simulink model "dcm2quat_test"  (R2018b)
settings: Solver=VariableStepAuto  StartTime=0.0  StopTime=10.0  RelTol=1e-3
libraries: sharedtransform x1
settings Model: Creator=taylorreynolds  LastModifiedBy=taylorreynolds

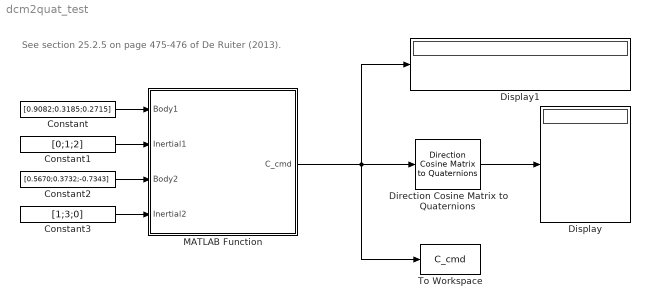
== system dcm2quat_test ==
  note: See section 25.2.5 on page 475-476 of De Ruiter (2013).
  Constant : Constant  Value=[0.9082;0.3185;0.2715]
  Constant1 : Constant  Value=[0;1;2]
  Constant2 : Constant  Value=[0.5670;0.3732;-0.7343]
  Constant3 : Constant  Value=[1;3;0]
  Direction Cosine Matrix to Quaternions : sharedtransform/Direction Cosine Matrix  to Quaternions  aMode=0  action=Error  tolerance=eps(2)
      settings: SourceProductName=Aerospace Blockset  SourceProductBaseCode=AE
  Display : Display
  Display1 : Display
  MATLAB Function : MATLAB Function  TreatAsAtomicUnit=on
  To Workspace : ToWorkspace  VariableName=C_cmd  SampleTime=-1
      settings: MaxDataPoints=1
  wires:
  MATLAB Function/1(C_cmd) -> To Workspace/1, Display1/1, Direction Cosine Matrix to Quaternions/1
  Direction Cosine Matrix to Quaternions/1 -> Display/1
  Constant/1 -> MATLAB Function/1(Body1)
  Constant3/1 -> MATLAB Function/4(Inertial2)
  Constant2/1 -> MATLAB Function/3(Body2)
  Constant1/1 -> MATLAB Function/2(Inertial1)

== matlab function dcm2quat_test/MATLAB Function ==
  data: Body1 input; C_cmd output; Inertial1 input; Body2 input; Inertial2 input
function C_cmd  = align_vecs(Body1, Inertial1, Body2, Inertial2) 
    
    % Body
    Body1 = Body1./norm(Body1); %takes precident
    Body2 = Body2./norm(Body2);
    Xtb = Body1;
    Ytb = cross(Body1,Body2);
    Ytb = Ytb./norm(Ytb);%/norm(cross(Body1,Body2));
    Ztb = cross(Body1,Ytb);
    Ztb = Ztb./norm(Ztb);%/norm(cross(Body1,Ytb));
    
    % Inertial
    Inertial1 = Inertial1./norm(Inertial1); % set to align with B1
    Inertial2 = Inertial2./norm(Inertial2); % set to partially align with B2
    Xti = Inertial1;
    Yti = cross(Inertial1,Inertial2);
    Yti = Yti./norm(Yti);%/norm(cross(Inertial1,Inertial2));
    Zti = cross(Inertial1,Yti);
    Zti = Zti./norm(Zti);%/norm(cross(Inertial1,Yti));
    
    % Stack vectors
    Cb  = [Xtb, Ytb, Ztb];
    Ci  = [Xti, Yti, Zti];
    
    % Commanded DCM ( body to inertial )
    C_cmd   = Cb*Ci';

end
